simulink model "classpractice"  (R2021a)
settings: Solver=VariableStepAuto  StartTime=0.0  StopTime=10.0  RelTol=1e-3
libraries: spsIGBTDiodeLib x4, spsCurrentMeasurementLib x2, spsVoltageMeasurementLib x2, spsSeriesRLCBranchLib x1, spsTriangleGeneratorLib x1, spsDCVoltageSourceLib x1, spspowerguiLib x1
settings Model: Creator=User  LastModifiedBy=User

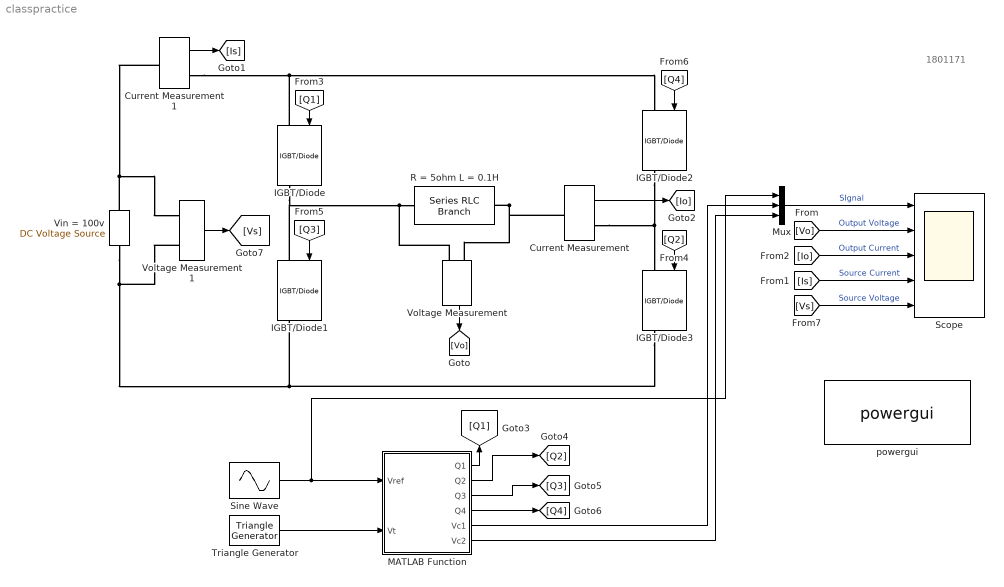
== system classpractice ==
  note: 1801171
  Current Measurement : spsCurrentMeasurementLib/Current Measurement  PhasorSimulation=off  OutputType=Complex  PSBequivalent=0
  Current Measurement1 : spsCurrentMeasurementLib/Current Measurement  PhasorSimulation=off  OutputType=Complex  PSBequivalent=0
  IGBT/Diode{,1..3} (4 alike) : spsIGBTDiodeLib/IGBT//Diode  Ron=1e-3  Rs=1e5  Cs=inf  Measurements=on
  MATLAB Function : MATLAB Function  TreatAsAtomicUnit=on
  Mux : Mux  Inputs=3
  R = 5ohm L = 0.1H : spsSeriesRLCBranchLib/Series RLC Branch  LConnTagsString=__new0  RConnTagsString=__new0  BranchType=RL  Resistance=5  Inductance=100e-3  SetiL0=off  InitialCurrent=0  Capacitance=1e-6  Setx0=off  InitialVoltage=0  Measurements=None
  Scope : Scope  NumInputPorts=5
  Sine Wave : Sin  Amplitude=15  Frequency=2*pi*50  SampleTime=0
  Triangle Generator : spsTriangleGeneratorLib/Triangle Generator  Freq=1000  Phase=0  Ts=0
  Vin = 100v : spsDCVoltageSourceLib/DC Voltage Source  Amplitude=100  Measurements=None
  Voltage Measurement : spsVoltageMeasurementLib/Voltage Measurement  PhasorSimulation=off  OutputType=Complex  PSBequivalent=0
  Voltage Measurement1 : spsVoltageMeasurementLib/Voltage Measurement  PhasorSimulation=off  OutputType=Complex  PSBequivalent=0
  powergui : spspowerguiLib/powergui  Priority=1  SimulationMode=Discrete  SampleTime=0.5e-6  frequency=60  Iterations=50  frequencyindice=0  Pbase=100e6  ErrMax=1e-4  UnitsV=kV  UnitsW=MW  buscounter=0  FunctionMessages=off  echomessages=off  EnableUseOfTLC=off  CurrentSourceSwitches=off  DisableSnubberDevices=off  DisableRonSwitches=off  DisableVfSwitches=off  DisplayEquations=off  AutomaticDiscreteSolvers=off  SolverType=Tustin/Backward Euler (TBE)  Interpol=off  ExternalGateDelay=off  methode=off  Ts=100  x0status=blocks  SPID=on  SwTol=0  HookPort=off  NonlinearTolerance=1e-4  nMaxIteration=100  ContinueOnMaxIteration=off  RestoreLinks=warning  ResistiveCurrentMeasurement=off  Frange=[0:2:500]  Ylog=off  Xlog=on  ShowGrid=off  save=off  variable=ZData  structure=0  ZoomFFT=off  StartTime=0.0  cycles=1  DisplayStyle=1  fundamental=60  FreqAxis=off  MaxFrequency=1000  frequencyindicesteady=1  RmsSteady=1  display=off
  wires:
  MATLAB Function/4(Q4) -> [Q4]
  Voltage Measurement1/1 -> [Vs]
  MATLAB Function/1(Q1) -> [Q1]
  [Vs] -> Scope/5  "Source Voltage"
  Current Measurement1/1 -> [Is]
  [Q3] -> IGBT/Diode1/1
  [Q4] -> IGBT/Diode2/1
  [Q2] -> IGBT/Diode3/1
  [Io] -> Scope/3  "Output Current"
  [Is] -> Scope/4  "Source Current"
  Mux/1 -> Scope/1  "SIgnal"
  [Vo] -> Scope/2  "Output Voltage"
  MATLAB Function/2(Q2) -> [Q2]
  Voltage Measurement/1 -> [Vo]
  MATLAB Function/5(Vc1) -> Mux/2
  Current Measurement/1 -> [Io]
  MATLAB Function/3(Q3) -> [Q3]
  MATLAB Function/6(Vc2) -> Mux/3
  [Q1] -> IGBT/Diode/1
  Triangle Generator/1 -> MATLAB Function/2(Vt)
  Sine Wave/1 -> Mux/1, MATLAB Function/1(Vref)
  connections:
  Current Measurement1/LConn1 -- Vin = 100v/RConn1 -- Voltage Measurement1/LConn1
  Vin = 100v/LConn1 -- IGBT/Diode3/RConn1 -- IGBT/Diode1/RConn1 -- Voltage Measurement1/LConn2
  IGBT/Diode/LConn1 -- Current Measurement1/RConn1 -- IGBT/Diode2/LConn1
  R = 5ohm L = 0.1H/RConn1 -- Current Measurement/LConn1 -- Voltage Measurement/LConn2
  R = 5ohm L = 0.1H/LConn1 -- IGBT/Diode/RConn1 -- IGBT/Diode1/LConn1 -- Voltage Measurement/LConn1
  Current Measurement/RConn1 -- IGBT/Diode2/RConn1 -- IGBT/Diode3/LConn1

== matlab function classpractice/MATLAB Function ==
  data: Vref input; Q1 output; Vt input; Q2 output; Q3 output; Q4 output; Vc1 output; Vc2 output
function [Q1 ,Q2 ,Q3 ,Q4,Vc1,Vc2] = pulse(Vref, Vt)
Vc1 = (Vt+1)*0.5;
Vc2 = (Vt-1)*0.5;
if Vref>0
    if Vref >= Vc1
        Q1=1;
        Q2=1;
        Q3=0;
        Q4=0;
    else
        Q1=1;
        Q2=0;
        Q3=0;
        Q4=1;
    end
elseif Vref<0
    if Vref<=Vc2
        Q1=0;
        Q2=0;
        Q3=1;
        Q4=1;
    else
        Q1=0;
        Q2=1;
        Q3=1;
        Q4=0;
    end
else
    Q1=0;
    Q2=0;
    Q3=0;
    Q4=0;
end
end
